simulink model "simone_org"  (Simulink 10.0)
settings: Solver=VariableStepAuto  StartTime=0.0  StopTime=10.0  RelTol=1e-3
undefined symbols (not defined in the file): aNoisePower, D1D, D1N, D2D, D2N, inputTorque, l, m1, m2, thetaDNoisePower, Ts
libraries: simulink x4
settings Model: Creator=rosen  LastModifiedBy=annonymous
settings DataIOCC: SaveFormat=Dataset
settings OptimizationCC: LifeSpan=auto
settings DebuggingCC: UnderspecifiedInitializationDetection=Simplified  MergeDetectMultiDrivingBlocksExec=error  SFUnexpectedBacktrackingDiag=error  SFNoUnconditionalDefaultTransitionDiag=error  SFExecutionAtInitializationDiag=warning
settings HardwareCC: ProdBitPerPointer=64  ProdBitPerSizeT=64  ProdBitPerPtrDiffT=64  ProdLargestAtomicFloat=Float  ProdIntDivRoundTo=Zero  ProdEndianess=LittleEndian  ProdWordSize=64  ProdHWDeviceType=Intel->x86-64 (Windows64)
settings ModelReferenceCC: PropagateSignalLabelsOutOfModel=on
settings GRTTargetCC: TargetLangStandard=C99 (ISO)  CombineOutputUpdateFcns=on  GRTInterface=off
settings ConfigComp: CovMetricSettings=dwe  CovHtmlReporting=off  CovSaveCumulativeToWorkspaceVar=off  CovSaveSingleToWorkspaceVar=off

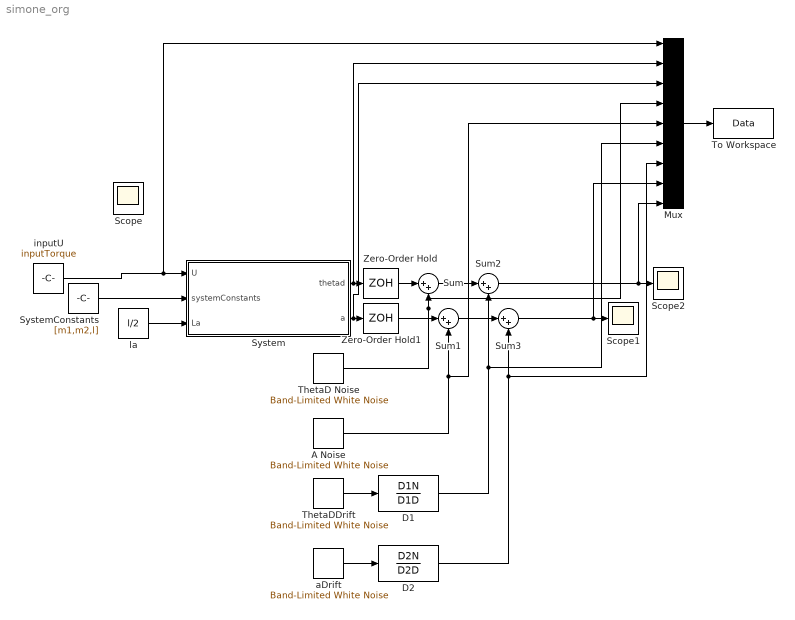
== system simone_org ==
  A Noise : simulink/Sources/Band-Limited White Noise  Cov=[aNoisePower]  Ts=Ts  seed=[23341]
  D1 : DiscreteTransferFcn  Numerator=D1N  Denominator=D1D  SampleTime=Ts
  D2 : DiscreteTransferFcn  Numerator=D2N  Denominator=D2D  SampleTime=Ts
  Mux : Mux  Inputs=9
  Scope1 : Scope
  Scope2 : Scope
  Sum{,1..3} (4 alike) : Sum  Inputs=|++
  System : Subsystem
  SystemConstants : Constant  Value=[m1,m2,l]
  ThetaD Noise : simulink/Sources/Band-Limited White Noise  Cov=[thetaDNoisePower]  Ts=Ts  seed=[23341]
  ThetaDDrift : simulink/Sources/Band-Limited White Noise  Cov=[0.1]  Ts=Ts  seed=[23341]
  To Workspace : ToWorkspace  VariableName=Data  SaveFormat=Timeseries  SampleTime=-1
  Zero-Order Hold : ZeroOrderHold  SampleTime=Ts
  Zero-Order Hold1 : ZeroOrderHold  SampleTime=Ts
  aDrift : simulink/Sources/Band-Limited White Noise  Cov=[0.1]  Ts=Ts  seed=[23341]
  inputU : Constant  Value=inputTorque
  la : Constant  Value=l/2
  Scope : Scope
  wires:
  SystemConstants/1 -> System/2(systemConstants)
  la/1 -> System/3(La)
  inputU/1 -> Mux/1, System/1(U)
  ThetaDDrift/1 -> D1/1
  aDrift/1 -> D2/1
  System/1("thetad ") -> Mux/2, Zero-Order Hold/1
  System/2(a) -> Mux/3, Zero-Order Hold1/1
  Zero-Order Hold/1 -> Sum/1
  Zero-Order Hold1/1 -> Sum1/1
  Sum/1 -> Sum2/1
  Sum1/1 -> Sum3/1
  Sum2/1 -> Mux/9, Scope2/1
  Sum3/1 -> Mux/8, Scope1/1
  ThetaD Noise/1 -> Mux/4, Sum/2
  A Noise/1 -> Mux/5, Sum1/2
  D1/1 -> Mux/6, Sum2/2
  D2/1 -> Mux/7, Sum3/2
  Mux/1 -> To Workspace/1

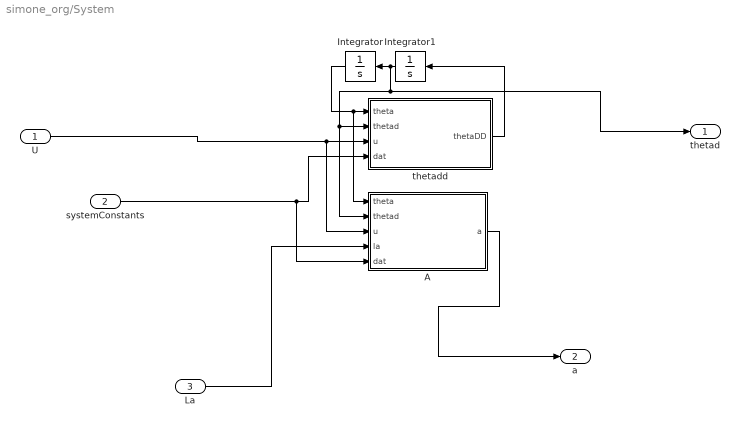
== system simone_org/System ==
  U : Inport
  systemConstants : Inport  Port=2
  La : Inport  Port=3
  A : MATLAB Function  TreatAsAtomicUnit=on
  Integrator : Integrator
  Integrator1 : Integrator
  thetadd : MATLAB Function  TreatAsAtomicUnit=on
  "thetad " : Outport
  a : Outport  Port=2
  wires:
  thetadd/1(thetaDD) -> Integrator1/1
  Integrator/1 -> A/1(theta), thetadd/1(theta)
  La/1 -> A/4(la)
  U/1 -> A/3(u), thetadd/3(u)
  systemConstants/1 -> A/5(dat), thetadd/4(dat)
  Integrator1/1 -> "thetad "/1, thetadd/2(thetad), A/2(thetad), Integrator/1
  A/1(a) -> a/1

== matlab function System/A ==
  data: theta input double; thetad input double; u input double; a output double; la input double; dat input double
function a = A(theta,thetad,u,la,dat)
m1 = dat(1);
m2 = dat(2);
l = dat(3);

one = (l-la)/l;
two = (cos(theta)-m1*l*cos(theta)*thetad^2*sin(theta))*u;
three = m1+m2-m1*cos(theta)^2;
four = (m1+m2)*9.81*sin(theta);

a = one*(two/three + four/three);

end

== matlab function System/thetadd ==
  data: theta input double; thetad input double; u input double; thetaDD output double; dat input double
function thetaDD = thetadd(theta, thetad,u,  dat)

m1 = dat(1);
m2 = dat(2);
l = dat(3);

a = (9.81*(m1+m2)-m1*l*cos(theta)*thetad^2)*sin(theta);
b = cos(theta)*u;
c = l*(m1+m2-m1*cos(theta)^2);

thetaDD = (a+b)/c;

end
